simulink model "SMC_test"  (R2023a)
settings: Solver=VariableStepAuto  StartTime=0.0  StopTime=20  RelTol=1e-3
settings Model: Creator=edzel  LastModifiedBy=edzel

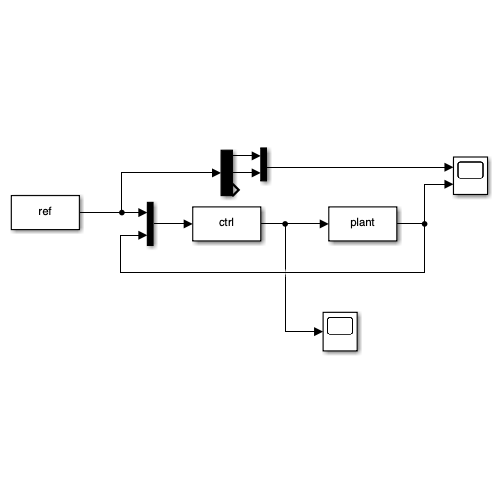
[thumbnail: Simulink's stored preview of the top-level diagram]
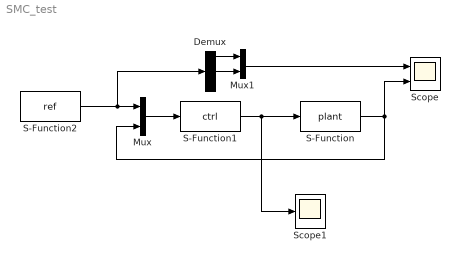
== system SMC_test ==
  Demux : Demux  Outputs=3
  Mux : Mux  Inputs=2
  Mux1 : Mux  Inputs=2
  S-Function : S-Function  FunctionName=plant  Parameters=pa  SFunctionDeploymentMode=off  EnableBusSupport=off
  S-Function1 : S-Function  FunctionName=ctrl  Parameters=pa  SFunctionDeploymentMode=off  EnableBusSupport=off
  S-Function2 : S-Function  FunctionName=ref  Parameters=pa  SFunctionDeploymentMode=off  EnableBusSupport=off
  Scope : Scope  NumInputPorts=2
  Scope1 : Scope
  wires:
  S-Function1/1 -> Scope1/1, S-Function/1
  Mux/1 -> S-Function1/1
  S-Function2/1 -> Demux/1, Mux/1
  S-Function/1 -> Scope/2, Mux/2
  Demux/1 -> Mux1/1
  Demux/2 -> Mux1/2
  Mux1/1 -> Scope/1
